simulink subsystem "Kalman_Filter"  (R2022b)
settings: Solver=VariableStepAuto  StartTime=0.0  StopTime=10.0  RelTol=1e-3
values from neighbouring files (symbols this model uses):
  A = [0, motor.gearbox, 0; 0, -motor.B/motor.J, motor.Kphi/motor.J; 0, -motor.Kphi/motor.La, -motor.Ra/motor.La]    [Kalman_Filter.m]    (also in Lqr_Controller_Tune.m = [; Model_Parameters.m = [0, motor.gearbox, 0; 0, -1/motor.Tm, motor.Kphi/motor.J; 0,; Observer_Tune.m = [0 motor.gearbox 0; 0 -motor.B/motor.J motor.Kphi/motor.J; 0)
  Ak = [  0   motor.gearbox           0           0 ... (first row only)    [Kalman_Tune.m]
  B = [0; 0; 1/motor.La]    [Kalman_Filter.m]    (also in Lqr_Controller_Tune.m; Model_Parameters.m; Observer_Tune.m)
  Bk = [0; 0; 0; 1/motor.La]    [Kalman_Tune.m]
  C = [0, 0, 1; 1, 0, 0]    [Kalman_Filter.m]    (also in Lqr_Controller_Tune.m = [1 0 0; 0 0 1]; Model_Parameters.m = [1 0 0; 0 0 1]; Observer_Tune.m = [1 0 0; 0 0 1])
  Ck = [1 0 0 0; 0 0 0 1]    [Kalman_Tune.m]
  Dk = zeros(2, 1)    [Kalman_Tune.m]
  Q = 0*eye(3)    [Kalman_Filter.m]    (also in Kalman_Tune.m = diag([0, 1, motor.tau, 0]); Lqr_Controller_Tune.m = C'*C)
  R = eye(2)    [Kalman_Filter.m]    (also in Kalman_Tune.m = diag([AS5600.q_rad^2/12, 1]); Lqr_Controller_Tune.m = 0.0002)
undefined symbols (not defined in the file or in its folder): bridge, Discrete, motor, Time, uc
libraries: ctrlSharedLib x1, dspinverses x1
settings Model: Creator=gotta  LastModifiedBy=gotta

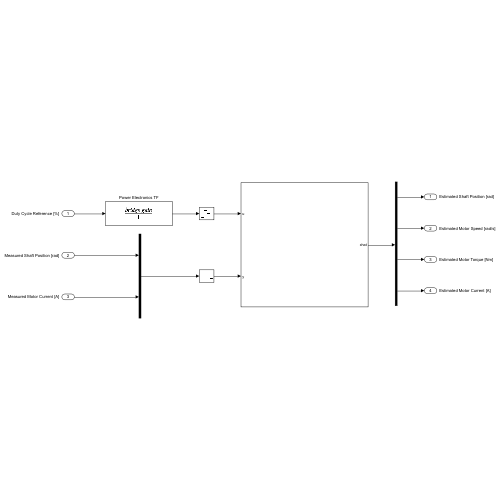
[thumbnail: Simulink's stored preview of the top-level diagram]
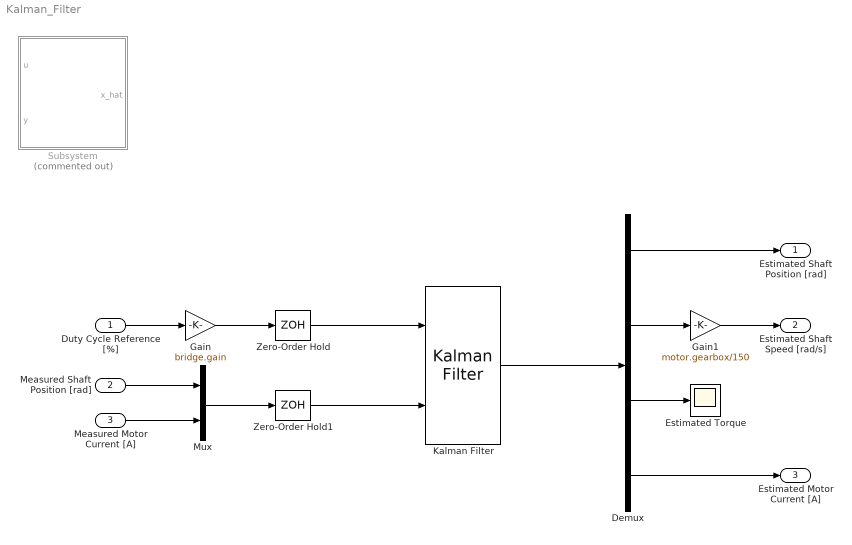
== system Kalman_Filter ==
  Duty Cycle Reference [%] : Inport
  Measured Shaft Position [rad] : Inport  Port=2
  Measured Motor Current [A] : Inport  Port=3
  Demux : Demux
  Estimated Torque : Scope
  Gain : Gain  Gain=bridge.gain
  Gain1 : Gain  Gain=motor.gearbox/150
  Kalman Filter : ctrlSharedLib/Kalman Filter  TimeDomain=Discrete-Time  UseCurrentEstimator=on  ModelSource=Individual A, B, C, D matrices  ModelSourceVariable=ss(0.95,1,1,0,1)  A=Ak  B=Bk  C=Ck  D=Dk  NumberOfStates=1  NumberOfInputs=1  NumberOfOutputs=1  InitialEstimateSource=Dialog  X0=0  P0=10  UseK=off  UseGH=off  NumberOfProcessNoiseInputs=1  G=1  TimeInvariantG=on  H=0  TimeInvariantH=on  Q=Q  TimeInvariantQ=on  R=R  TimeInvariantR=on  N=0  TimeInvariantN=on  AddInputPort=on  AddEnablePort=off  OutputEstimatedY=off  OutputP=off  Ts=uc.Ts
  Mux : Mux  Inputs=2
  Subsystem : Subsystem  Commented=on  mask{Value_A=A, Value_B=B, Value_C=C, Value_Q=Q, Value_R=R}
      mask prompts: Value_A "A"; Value_B "B"; Value_C "C"; Value_Q "Q"; Value_R "R"
      mask TypeOptions Value_A: A/Value
      mask TypeOptions Value_B: B/Value
      mask TypeOptions Value_C: C/Value
      mask TypeOptions Value_Q: Q/Value
      mask TypeOptions Value_R: R/Value
  Zero-Order Hold : ZeroOrderHold  SampleTime=uc.Ts
  Zero-Order Hold1 : ZeroOrderHold  SampleTime=uc.Ts
  Estimated Shaft Position [rad] : Outport
  Estimated Shaft Speed [rad/s] : Outport  Port=2
  Estimated Motor Current [A] : Outport  Port=3
  wires:
  Duty Cycle Reference [%]/1 -> Gain/1
  Demux/1 -> Estimated Shaft Position [rad]/1
  Demux/2 -> Gain1/1
  Measured Motor Current [A]/1 -> Mux/2
  Measured Shaft Position [rad]/1 -> Mux/1
  Mux/1 -> Zero-Order Hold1/1
  Gain/1 -> Zero-Order Hold/1
  Demux/4 -> Estimated Motor Current [A]/1
  Zero-Order Hold/1 -> Kalman Filter/1
  Zero-Order Hold1/1 -> Kalman Filter/2
  Kalman Filter/1 -> Demux/1
  Gain1/1 -> Estimated Shaft Speed [rad/s]/1
  Demux/3 -> Estimated Torque/1

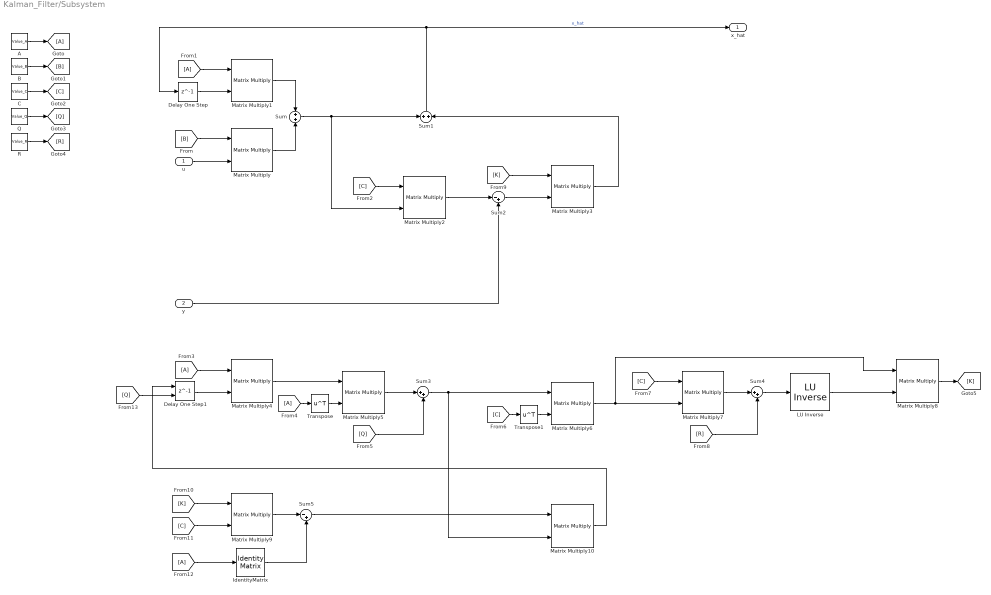
== system Kalman_Filter/Subsystem ==
  u : Inport
  y : Inport  Port=2
  " LU Inverse" : dspinverses/ LU Inverse
  A : Constant  Value=Value_A
  B : Constant  Value=Value_B
  C : Constant  Value=Value_C
  Delay One Step : Delay  DelayLength=1  SampleTime=uc.Ts
  Delay One Step1 : Delay  DelayLength=1  InitialConditionSource=Input port  InitialCondition=Q  SampleTime=uc.Ts
      settings: InputPortMap=u0,p4
  From{1,3..4,12} (4 alike) : From
  Goto : Goto
  IdentityMatrix : IdentityMatrix  InheritOutputPortAttributes=on
  Matrix Multiply{,1..10} (11 alike) : Product  Multiplication=Matrix(*)
  Q : Constant  Value=Value_Q
  R : Constant  Value=Value_R
  Sum : Sum  Inputs=+|+
  Sum1 : Sum  Inputs=+|+
  Sum2 : Sum  Inputs=|-+
  Sum3 : Sum  Inputs=|++
  Sum4 : Sum  Inputs=|++
  Sum5 : Sum  Inputs=|-+
  Transpose : Math  Operator=transpose
  Transpose1 : Math  Operator=transpose
  x_hat : Outport
  wires:
  [Q] -> Delay One Step1/2
  From12/1 -> IdentityMatrix/1
  u/1 -> Matrix Multiply/2
  [C] -> Matrix Multiply9/2
  Matrix Multiply8/1 -> [K]
  Transpose1/1 -> Matrix Multiply6/2
  B/1 -> [B]
  Matrix Multiply2/1 -> Sum2/1
  IdentityMatrix/1 -> Sum5/2
  Matrix Multiply3/1 -> Sum1/2
  Sum4/1 -> " LU Inverse"/1
  Delay One Step/1 -> Matrix Multiply1/2
  Sum/1 -> Sum1/1, Matrix Multiply2/2
  [B] -> Matrix Multiply/1
  Matrix Multiply4/1 -> Matrix Multiply5/1
  From3/1 -> Matrix Multiply4/1
  [C] -> Transpose1/1
  [C] -> Matrix Multiply2/1
  From4/1 -> Transpose/1
  From1/1 -> Matrix Multiply1/1
  [K] -> Matrix Multiply9/1
  Matrix Multiply9/1 -> Sum5/1
  Sum2/1 -> Matrix Multiply3/2
  R/1 -> [R]
  Matrix Multiply1/1 -> Sum/1
  Matrix Multiply5/1 -> Sum3/1
  y/1 -> Sum2/2
  Sum3/1 -> Matrix Multiply6/1, Matrix Multiply10/2
  [K] -> Matrix Multiply3/1
  Matrix Multiply10/1 -> Delay One Step1/1
  C/1 -> [C]
  Sum5/1 -> Matrix Multiply10/1
  " LU Inverse"/1 -> Matrix Multiply8/2
  A/1 -> Goto/1
  [C] -> Matrix Multiply7/1
  [R] -> Sum4/2
  [Q] -> Sum3/2
  Matrix Multiply6/1 -> Matrix Multiply7/2, Matrix Multiply8/1
  Q/1 -> [Q]
  Transpose/1 -> Matrix Multiply5/2
  Matrix Multiply/1 -> Sum/2
  Matrix Multiply7/1 -> Sum4/1
  Sum1/1 -> Delay One Step/1, x_hat/1  "x_hat"
  Delay One Step1/1 -> Matrix Multiply4/2
